simulink model "ssc_airvtol_elec_battery"  (R2026a)
settings: Solver=daessc  StopTime=2000  AbsTol=1e-3  EnableMultiTasking=on
PreLoadFcn:
  | ssc_airvtol_elec_default_params
  | battery_capacity = 180;battery_pdensity = 240;payload_mass_workspace = 80;
PostLoadFcn:
  | warning('off','physmod:common:gl:sli:rtp:InvalidNonValueReference');
  | warning off Simulink:Engine:SortDiscontinuityInAlgLoop
model workspace (MATLAB code in the model file):
  | v0                 = 0; % Initial vehicle speed
  | wheel_radius = 0.15; % Wheel radius
  | k                   = 1e-2; % Motor losses (W/(N*M)^2)
  | t_torque        = 0.02; % Electric motor time constant
  | rpm0             = 2000; % Engine initial speed demand
undefined symbols (not defined in the file): battery_vnom, propeller_num
libraries: fl_lib x49, nesl_utility x13, ee_lib x12, ssc_airvtol_components x11, sdl_lib x8, simulink x6, batteryecm_lib x2, pack_5p48s8p_Thr_library x2, pack_5p48s8p_1g10g1_5g1g5_Thr_library x1, pack_5p48s8p_1g10g1_Iso_library x1, pack_5p48s8p_1g10g1_Thr_library x1, pack_5p48s8p_4g4g4_Iso_library x1
(part 1 of 2)
CloseFcn:
  | try,close(h1_ssc_airvtol_elec),end
  | clear h1_ssc_airvtol_elec
  | try,close(h2_ssc_airvtol_elec),end
  | clear h2_ssc_airvtol_elec
  | try,close(h3_ssc_airvtol_elec),end
  | clear h3_ssc_airvtol_elec
  | try,close(h4_ssc_airvtol_elec),end
  | clear h4_ssc_airvtol_elec
  | try,close(h5_ssc_airvtol_elec),end
  | clear h5_ssc_airvtol_elec
  | try,close(h6_ssc_airvtol_elec),end
  | clear h6_ssc_airvtol_elec
  | try,close(h7_ssc_airvtol_elec),end
  | clear h7_ssc_airvtol_elec
  | try,close(h8_ssc_airvtol_elec),end
  | clear h8_ssc_airvtol_elec
  | try,close(h9_ssc_airvtol_elec),end
  | clear h9_ssc_airvtol_elec
  | try,close(h10_ssc_airvtol_elec),end
  | clear h10_ssc_airvtol_elec
  | 
  | clear simlog_ssc_airvtol_elec
  | clear logsout_ssc_airvtol_elec
Description:
  | Electric Aircraft (VTOL) Battery Design Exploration
  | 
  | Copyright 2022-2026 The MathWorks, Inc.
settings Model: FPTRunName=Active  Creator=MathWorks  LastModifiedBy=smiller
settings DataIOCC: InitialState=xBaseline  SaveOperatingPoint=on  SignalLoggingSaveFormat=ModelDataLogs  SignalLoggingName=logsout_ssc_airvtol_elec
settings DebuggingCC: UnderspecifiedInitializationDetection=Classic  PregeneratedLibrarySubsystemCodeDiagnostic=none
settings HardwareCC: ProdHWDeviceType=32-bit Generic
settings GRTTargetCC: CombineOutputUpdateFcns=off  GRTInterface=on
settings SimscapeCC: SimscapeNormalizeSystem=off  SimscapeNominalValues="[{\"value\":\"1\",\"unit\":\"A\"},{\"value\":\"1\",\"unit\":\"bar\"},{\"value\":\"1\",\"unit\":\"cm^2\"},{\"value\":\"1\",\"unit\":\"cm^3/s\"},{\"value\":\"1\",\"unit\":\"kJ/kg\"},{\"value\":\"1\",\"unit\":\"kW\"},{\"value\":\"1\",\"unit\":\"l\"},{\"value\":\"1\",\"unit\":\"N\"},{\"value\":\"1\",\"unit\":\"N*m\"},{\"value\":\"1\",\"unit\":\"V\"}]"  SimscapeLogSimulationStatistics=on  SimscapeLogName=simlog_ssc_airvtol_elec

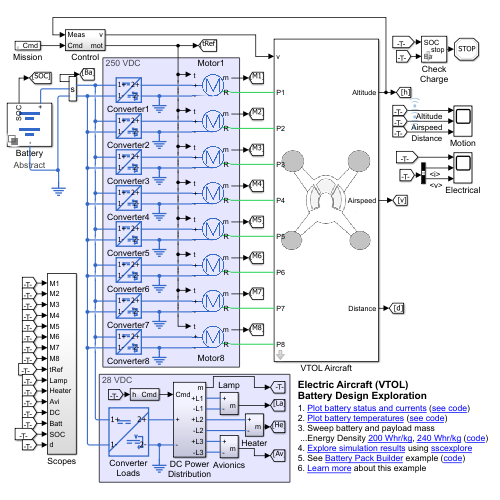
[thumbnail: Simulink's stored preview of the top-level diagram]
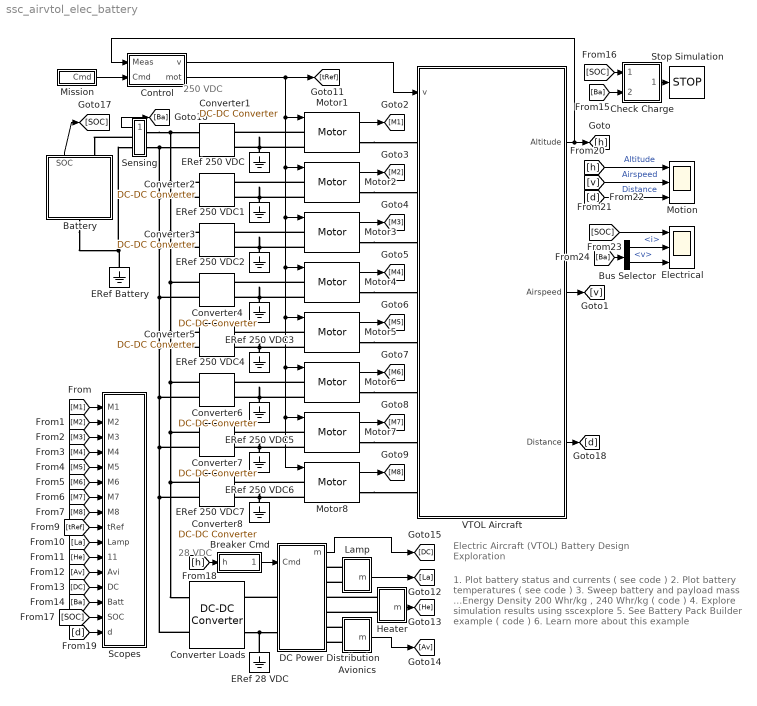
== system ssc_airvtol_elec_battery ==
  note: 250 VDC
  note: 28 VDC
  note: Electric Aircraft (VTOL)
      | Battery Design Exploration
  note: 1. Plot battery status and currents ( see code )
      | 2. Plot battery temperatures ( see code )
      | 3. Sweep battery and payload mass
      | ...Energy Density 200 Whr/kg , 240 Whr/kg ( code )
      | 4. Explore simulation results using sscexplore
      | 5. See Battery Pack Builder example ( code )
      | 6. Learn more about this example
  Avionics : Subsystem
  Battery : Subsystem  Variant=on  VariantControlMode=label  VariantControl=Equal_Iso  LabelModeActiveChoice=Abstract
      settings: AttributesFormatString=%<LabelModeActiveChoice>
  Breaker Cmd : Subsystem
  Bus Selector : BusSelector  OutputSignals=i,v
  Check Charge : Subsystem  mask{q_battery_limit=0.3}
      mask prompts: q_battery_limit "Battery charge lower limit (A*hr)"
  Control : Subsystem
  Converter Loads : ee_lib/Semiconductors & Converters/Converters/DC-DC Converter  Vref_option=ee.enum.converters.voltageref.internal  v_ref=28 V  P_rated=4 kW  droop_enabled=true  droop_param=ee.enum.converters.droop.value  droop=0.01 V/A  droop_percent=2  Vref_droop=10 V  reversible=ee.enum.converters.directionality.unidirectional  G_diode=1e-8 1/Ohm  P_fixed=100 W  losses_option=ee.enum.converters.lossesOption.proportionalToSquaredCurrent  eff_rated=97  tableOption=ee.enum.converters.lossTableOption.current  i_eff_vec=[1, 2, 3, 4] A  v_eff_vec=[15, 30, 45] V  eff_vec=[90, 80, 70, 60]  eff_2D_table=[90, 85, 80; 80, 75, 70; 70, 65, 60; 60, 55, 50]  model_dynamics=ee.enum.converters.dynamics.yes  tau=0.02 s  v_ini=28 V  v1_min=1 V  R1=1000 Ohm  R2=1000 Ohm  T_eff_vec=[280, 300, 320] K  eff_3D_table=repmat([66; 76; 80; 74], 1, 3, 3)  thermal_mass=100 J/K  initial_temperature=298.15 K
  Converter{1..8} (8 alike) : ee_lib/Semiconductors & Converters/Converters/DC-DC Converter  Vref_option=ee.enum.converters.voltageref.internal  v_ref=250 V  P_rated=1200 kW  droop_enabled=true  droop_param=ee.enum.converters.droop.value  droop=0.001 V/A  droop_percent=2  Vref_droop=10 V  reversible=ee.enum.converters.directionality.bidirectional  G_diode=1e-8 1/Ohm  P_fixed=100 W  losses_option=ee.enum.converters.lossesOption.proportionalToSquaredCurrent  eff_rated=97  tableOption=ee.enum.converters.lossTableOption.current  i_eff_vec=[1, 2, 3, 4] A  v_eff_vec=[15, 30, 45] V  eff_vec=[90, 80, 70, 60]  eff_2D_table=[90, 85, 80; 80, 75, 70; 70, 65, 60; 60, 55, 50]  model_dynamics=ee.enum.converters.dynamics.yes  tau=0.02 s  v_ini=250 V  v1_min=1 V  R1=1000 Ohm  R2=1000 Ohm  T_eff_vec=[280, 300, 320] K  eff_3D_table=repmat([66; 76; 80; 74], 1, 3, 3)  thermal_mass=100 J/K  initial_temperature=298.15 K
  DC Power Distribution : Subsystem
  ERef 250 VDC{,1..7} (8 alike) : fl_lib/Electrical/Electrical Elements/Electrical Reference
  ERef 28 VDC : fl_lib/Electrical/Electrical Elements/Electrical Reference
  ERef Battery : fl_lib/Electrical/Electrical Elements/Electrical Reference
  Electrical : Scope  NumInputPorts=3
      settings: Title=Battery SOC  ActiveDisplayYMinimum=0.2125  ActiveDisplayYMaximum=1.0875  DataLoggingVariableName=ScopeData3
  Heater : Subsystem
  Lamp : Subsystem
  Mission : Subsystem  mask(Mission Parameters){t_climb=30, h_cruise=100}
      mask prompts: t_climb "Time to reach cruise height (sec)"; h_cruise "Cruise height (m)"
      mask help: Define mission parameters.
  Motion : Scope  NumInputPorts=3
      settings: ActiveDisplayYMinimum=-12.74881  ActiveDisplayYMaximum=114.73236
  Motor{1..8} (8 alike) : ssc_airvtol_components/Motor  SystemSampleTime=-1  VariantActivationTime=update diagram  EmptyChoice=off  PassThrough=off  PassThroughVariantControl=(default)  EmptyChoiceVariantControl=(default)  AllowFlexibleInterface=on  Latency=0  AutoFrameSizeCalculation=off
  Scopes : Subsystem
  Sensing : Subsystem
      mask Display: disp('s');
  Stop Simulation : Stop
  VTOL Aircraft : Subsystem  mask(VTOL Aircraft){battery_power_density=battery_pdensity, battery_voltage=battery_vnom, battery_capacity=battery_capacity, aircraft_mass=60, inertia_prop=0.09, D_prop=1.5, kt_const=0.15, kp_const=0.13, rho=1.225}
      mask prompts: battery_power_density "Power Density (W*hr/kg)"; battery_voltage "Voltage (V)"; battery_capacity "Capacity (A*hr)"; aircraft_mass "Chassis Mass (without battery) (kg)"; inertia_prop "Inertia (kg*m^2)"; D_prop "Diameter"; kt_const "Thrust coefficient, kT"; kp_const "Power coefficient, kP"; rho "Fluid density"
      mask help: Define parameters for airframe, including values to compute total mass and propeller characteristics.
      mask init:
      | battery_mass = battery_capacity*battery_voltage/battery_power_density;
      mask TypeOptions inertia_prop: Inertia1/inertia | Inertia2/inertia | Inertia3/inertia | Inertia4/inertia | Inertia5/inertia | Inertia6/inertia | Inertia7/inertia | Inertia8/inertia
      mask TypeOptions D_prop: Propeller 1/D | Propeller 2/D | Propeller 3/D | Propeller 4/D | Propeller 5/D | Propeller 6/D | Propeller 7/D | Propeller 8/D
      mask TypeOptions kt_const: Propeller 1/kt_const | Propeller 2/kt_const | Propeller 3/kt_const | Propeller 4/kt_const | Propeller 5/kt_const | Propeller 6/kt_const | Propeller 7/kt_const | Propeller 8/kt_const
      mask TypeOptions kp_const: Propeller 1/kp_const | Propeller 2/kp_const | Propeller 3/kp_const | Propeller 4/kp_const | Propeller 5/kp_const | Propeller 6/kp_const | Propeller 7/kp_const | Propeller 8/kp_const
      mask TypeOptions rho: Propeller 1/rho | Propeller 2/rho | Propeller 3/rho | Propeller 4/rho | Propeller 5/rho | Propeller 6/rho | Propeller 7/rho | Propeller 8/rho
      mask DialogControl Container4 Prompt: Electrical
      mask DialogControl Container5 Prompt: Mechanical
      mask DialogControl cont_prop Prompt: Propeller
      mask Display: image('ssc_airvtol_battery_chassis_IMAGE.png')
  wires:
  VTOL Aircraft/3(Distance) -> [d]
  Breaker Cmd/1(Cmd) -> DC Power Distribution/1(Cmd)
  Check Charge/1(stop) -> Stop Simulation/1
  Battery/1(SOC) -> [SOC]
  VTOL Aircraft/1(Altitude) -> Control/1(Meas), [h]
  Motor1/1 -> [M1]
  Motor2/1 -> [M2]
  Motor3/1 -> [M3]
  Motor4/1 -> [M4]
  Motor5/1 -> [M5]
  Motor6/1 -> [M6]
  Motor7/1 -> [M7]
  Motor8/1 -> [M8]
  Mission/1(Cmd) -> Control/2(Cmd)
  Control/2(mot) -> Motor8/1, Motor7/1, Motor6/1, Motor5/1, Motor4/1, Motor3/1, Motor2/1, Motor1/1, [tRef]
  Control/1(v) -> VTOL Aircraft/1(v)
  [M1] -> Scopes/1(M1)
  [M2] -> Scopes/2(M2)
  [M3] -> Scopes/3(M3)
  [M4] -> Scopes/4(M4)
  [M5] -> Scopes/5(M5)
  [M6] -> Scopes/6(M6)
  [M7] -> Scopes/7(M7)
  [M8] -> Scopes/8(M8)
  [tRef] -> Scopes/9(tRef)
  Lamp/1(m) -> [La]
  [La] -> Scopes/10(Lamp)
  Heater/1(m) -> [He]
  Avionics/1(m) -> [Av]
  [He] -> Scopes/11(Heater)
  [Av] -> Scopes/12(Avi)
  DC Power Distribution/1(m) -> [DC]
  [DC] -> Scopes/13(DC)
  Sensing/1(m) -> [Ba]
  [Ba] -> Scopes/14(Batt)
  [Ba] -> Check Charge/2(Ba)
  [SOC] -> Check Charge/1(SOC)
  [SOC] -> Scopes/15(SOC)
  VTOL Aircraft/2(Airspeed) -> [v]
  [h] -> Breaker Cmd/1(h)
  [h] -> Motion/1  "Altitude"
  [v] -> Motion/2  "Airspeed"
  [d] -> Motion/3  "Distance"
  [SOC] -> Electrical/1
  [Ba] -> Bus Selector/1
  Bus Selector/1 -> Electrical/2  "<i>"
  Bus Selector/2 -> Electrical/3  "<v>"
  [d] -> Scopes/16(d)
  connections:
  Motor1/RConn1 -- VTOL Aircraft/LConn1
  Motor1/LConn1 -- Converter1/RConn1
  DC Power Distribution/LConn1 -- Converter Loads/RConn1
  Heater/LConn1 -- DC Power Distribution/RConn3
  Lamp/LConn2 -- DC Power Distribution/RConn2
  Lamp/LConn1 -- DC Power Distribution/RConn1
  Heater/LConn2 -- DC Power Distribution/RConn4
  Converter Loads/RConn2 -- ERef 28 VDC/LConn1 -- DC Power Distribution/LConn2
  ERef 250 VDC/LConn1 -- Motor1/LConn2 -- Converter1/RConn2
  ERef Battery/LConn1 -- Battery/LConn1 -- Sensing/RConn2
  Avionics/LConn1 -- DC Power Distribution/RConn5
  Avionics/LConn2 -- DC Power Distribution/RConn6
  Sensing/LConn1 -- Converter2/LConn1 -- Converter3/LConn1 -- Converter4/LConn1 -- Converter5/LConn1 -- Converter6/LConn1 -- Converter7/LConn1 -- Converter8/LConn1 -- Converter Loads/LConn1 -- Converter1/LConn1
  Converter Loads/LConn2 -- Sensing/LConn2 -- Converter1/LConn2 -- Converter2/LConn2 -- Converter3/LConn2 -- Converter4/LConn2 -- Converter5/LConn2 -- Converter6/LConn2 -- Converter7/LConn2 -- Converter8/LConn2
  ERef 250 VDC1/LConn1 -- Motor2/LConn2 -- Converter2/RConn2
  Motor2/LConn1 -- Converter2/RConn1
  Motor2/RConn1 -- VTOL Aircraft/LConn2
  ERef 250 VDC2/LConn1 -- Motor3/LConn2 -- Converter3/RConn2
  Motor3/LConn1 -- Converter3/RConn1
  Motor3/RConn1 -- VTOL Aircraft/LConn3
  ERef 250 VDC3/LConn1 -- Motor4/LConn2 -- Converter4/RConn2
  Motor4/LConn1 -- Converter4/RConn1
  Motor4/RConn1 -- VTOL Aircraft/LConn4
  ERef 250 VDC4/LConn1 -- Motor5/LConn2 -- Converter5/RConn2
  Motor5/LConn1 -- Converter5/RConn1
  Motor5/RConn1 -- VTOL Aircraft/LConn5
  ERef 250 VDC5/LConn1 -- Motor6/LConn2 -- Converter6/RConn2
  Motor6/LConn1 -- Converter6/RConn1
  Motor6/RConn1 -- VTOL Aircraft/LConn6
  ERef 250 VDC6/LConn1 -- Motor7/LConn2 -- Converter7/RConn2
  Motor7/LConn1 -- Converter7/RConn1
  Motor7/RConn1 -- VTOL Aircraft/LConn7
  ERef 250 VDC7/LConn1 -- Motor8/LConn2 -- Converter8/RConn2
  Motor8/LConn1 -- Converter8/RConn1
  Motor8/RConn1 -- VTOL Aircraft/LConn8
  Sensing/RConn1 -- Battery/RConn1

== system ssc_airvtol_elec_battery/Avionics ==
  Electrical Power : ssc_airvtol_components/Motor/Electrical Power  SystemSampleTime=-1  VariantActivationTime=update diagram  EmptyChoice=off  PassThrough=off  PassThroughVariantControl=(default)  EmptyChoiceVariantControl=(default)  AllowFlexibleInterface=on  Latency=0  AutoFrameSizeCalculation=off
  Resistor : fl_lib/Electrical/Electrical Elements/Resistor  R=1.5 Ohm  i_specify=off  i_priority=None  i=0 A  i_nominal_specify=off  i_nominal_value=1  i_nominal_unit=A  v_specify=off  v_priority=None  v=0 V  v_nominal_specify=off  v_nominal_value=1  v_nominal_unit=V
  + : PMIOPort  Side=Left
  - : PMIOPort  Port=2  Side=Left
  Out Bus Element : Outport  PortName=m  Element=Pe
  Out Bus Element3 : Outport  PortName=m  Element=i
  wires:
  Electrical Power/2 -> Out Bus Element3/1
  Electrical Power/1 -> Out Bus Element/1
  connections:
  Electrical Power/LConn1 -- +/RConn1
  Resistor/LConn1 -- Electrical Power/RConn1
  Resistor/RConn1 -- Electrical Power/LConn2 -- -/RConn1

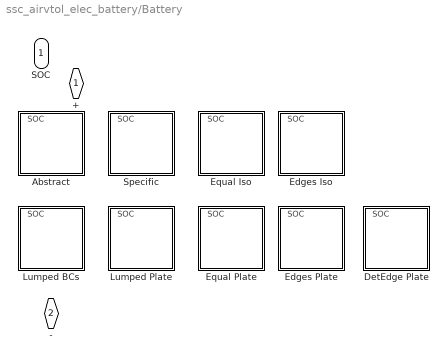
== system ssc_airvtol_elec_battery/Battery ==
  Abstract : Subsystem  VariantControl=Abstract
      mask Display: image('pack_abstract_IMAGE.png');
  DetEdge Plate : Subsystem  VariantControl=DetEdge_Plate
      mask Display: image('pack_5p48s8p_1g10g1_5g1g5_plate_IMAGE.png')
  Edges Iso : Subsystem  VariantControl=Edges_Iso
      mask Display: image('pack_5p48s8p_1g10g1_IMAGE.png')
  Edges Plate : Subsystem  VariantControl=Edges_Plate
      mask Display: image('pack_5p48s8p_1g10g1_plate_IMAGE.png')
  Equal Iso : Subsystem  VariantControl=Equal_Iso
      mask Display: image('pack_5p48s8p_4g4g4_IMAGE.png')
  Equal Plate : Subsystem  VariantControl=Equal_Plate
      mask Display: image('pack_5p48s8p_4g4g4_plate_IMAGE.png')
  Lumped BCs : Subsystem  VariantControl=Lumped_BCs
      mask Display: image('pack_5p48s8p_bcnd_IMAGE.png')
  Lumped Plate : Subsystem  VariantControl=Lumped_Plate
      mask Display: image('pack_5p48s8p_plate_IMAGE.png')
  Specific : Subsystem  VariantControl=Specific
      mask Display: image('pack_specific_IMAGE.png');
  + : PMIOPort  Side=Right
  - : PMIOPort  Port=2  Side=Left
  SOC : Outport

== system ssc_airvtol_elec_battery/Breaker Cmd ==
  h : Inport
  Avionics Breaker : Constant
  Heater Breaker OFF : Constant  Value=0
  Heater Breaker ON : Constant
  Lamp Breaker : Constant
  Mux1 : Mux  Inputs=3
  Switch : Switch  Threshold=50  ZeroCross=off  SaturateOnIntegerOverflow=off  InputSameDT=off
  Cmd : Outport  VectorParamsAs1DForOutWhenUnconnected=off
  wires:
  Mux1/1 -> Cmd/1
  Avionics Breaker/1 -> Mux1/3
  Lamp Breaker/1 -> Mux1/1
  Switch/1 -> Mux1/2
  h/1 -> Switch/2
  Heater Breaker ON/1 -> Switch/1
  Heater Breaker OFF/1 -> Switch/3

== system ssc_airvtol_elec_battery/Check Charge ==
  SOC : Inport
  In Bus Element : Inport  Port=2  PortName=Ba  Element=v
  In Bus Element1 : Inport  Port=2  PortName=Ba  Element=i
  Compare To Constant : simulink/Logic and Bit Operations/Compare To Constant  relop=<=  const=q_battery_limit  OutDataTypeStr=boolean
  Compare To Constant1 : simulink/Logic and Bit Operations/Compare To Constant  relop=<=  const=100  OutDataTypeStr=boolean
  Compare To Constant2 : simulink/Logic and Bit Operations/Compare To Constant  relop=>=  const=1000  OutDataTypeStr=boolean
  OR : Logic  Operator=OR  Inputs=3  IconShape=distinctive  AllPortsSameDT=off  OutDataTypeStr=boolean
  stop : Outport  VectorParamsAs1DForOutWhenUnconnected=off
  wires:
  Compare To Constant/1 -> OR/3
  In Bus Element/1 -> Compare To Constant1/1
  In Bus Element1/1 -> Compare To Constant2/1
  OR/1 -> stop/1
  Compare To Constant2/1 -> OR/2
  Compare To Constant1/1 -> OR/1
  SOC/1 -> Compare To Constant/1

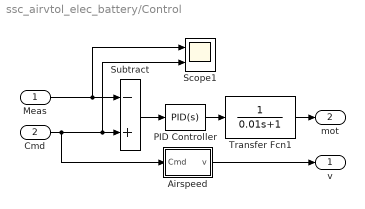
== system ssc_airvtol_elec_battery/Control ==
  Meas : Inport
  Cmd : Inport  Port=2
  Airspeed : Subsystem  mask(Conditions for Cruise){vCruise=28, vzth_Cruise=0.1, zth_Cruise=50}
      mask prompts: vCruise "Cruising speed (m/s)"; vzth_Cruise "Max vertical speed for cruise (m/s)"; zth_Cruise "Min altitude for cruise (m)"
      mask help: Define conditions for cruise speed.
  PID Controller : slpidlib/PID Controller  Controller=PID  Form=Parallel  TimeDomain=Continuous-time  UseExternalTs=off  SampleTime=-1  IntegratorMethod=Forward Euler  FilterMethod=Forward Euler  ControllerParametersSource=internal  P=1*10/2  I=0.08*10  UseKiTs=off  D=0.1*100  UseExternalDerivativeSource=off  N=100/100  UseFilter=on  TunerSelectOption=Transfer Function Based (PID Tuner App)  InitialConditionSource=internal  InitialConditionForIntegrator=0  InitialConditionForFilter=0  DifferentiatorICPrevScaledInput=0  ExternalReset=none  TrackingMode=off  Kt=1  LimitOutput=off  SatLimitsSource=internal  UpperSaturationLimit=inf  LowerSaturationLimit=-inf  LinearizeAsGain=on  AntiWindupMode=none  Kb=1  LimitIntegrator=off  UpperIntegratorSaturationLimit=inf  LowerIntegratorSaturationLimit=-inf  POutMin=[]  POutMax=[]  IOutMin=[]  IOutMax=[]  DOutMin=[]  DOutMax=[]  NOutMin=[]  NOutMax=[]  SumOutMin=[]  SumOutMax=[]  SaturationOutMin=[]  SaturationOutMax=[]  PParamMin=[]  PParamMax=[]  IParamMin=[]  IParamMax=[]  DParamMin=[]  DParamMax=[]  NParamMin=[]  NParamMax=[]  KbParamMin=[]  KbParamMax=[]  KtParamMin=[]  KtParamMax=[]  KbOutMin=[]  KbOutMax=[]  KtOutMin=[]  KtOutMax=[]  IntegratorOutMin=[]  IntegratorOutMax=[]  FilterOutMin=[]  FilterOutMax=[]  SumI1OutMin=[]  SumI1OutMax=[]  SumI2OutMin=[]  SumI2OutMax=[]  SumI3OutMin=[]  SumI3OutMax=[]  SumI4OutMin=[]  SumI4OutMax=[]  SumDOutMin=[]  SumDOutMax=[]  DifferentiatorOutMin=[]  DifferentiatorOutMax=[]  FilterDiffOutCoefMin=[]  FilterDiffOutCoefMax=[]  ReciprocalOutMin=[]  ReciprocalOutMax=[]  SumDenOutMin=[]  SumDenOutMax=[]  SumNumOutMin=[]  SumNumOutMax=[]  DivideOutMin=[]  DivideOutMax=[]  UdiffTsProdOutMin=[]  UdiffTsProdOutMax=[]  NTsProdOutMin=[]  NTsProdOutMax=[]  UintegralTsProdOutMin=[]  UintegralTsProdOutMax=[]  UngainTsProdOutMin=[]  UngainTsProdOutMax=[]  ClampingZeroOutDataTypeStr=Inherit: Inherit via back propagation  ClampingZeroOutMin=[]  ClampingZeroOutMax=[]  FilterDenConstantOutDataTypeStr=Inherit: Inherit via back propagation  FilterDenConstantOutMin=[]  FilterDenConstantOutMax=[]  PCopyOutDataTypeStr=Inherit: Inherit via back propagation  PCopyOutMin=[]  PCopyOutMax=[]  NCopyOutDataTypeStr=Inherit: Inherit via back propagation  NCopyOutMin=[]  NCopyOutMax=[]  IntegratorContinuousStateAttributes=''  IntegratorStateMustResolveToSignalObject=off  IntegratorRTWStateStorageClass=Auto  FilterContinuousStateAttributes=''  FilterStateMustResolveToSignalObject=off  FilterRTWStateStorageClass=Auto  ParallelPVariant=InternalParameters  IdealPVariant=Disabled  IVariant=InternalParameters  DVariant=InternalParameters  IntegratorVariant=Continuous  SatVariant=Disabled  AWVariant=Passthrough  PCopyVariant=Disabled  TRVariant=Disabled  FdbkBlocksVariant=Forward  IdealPFdbkVariant=Disabled  SatFdbkVariant=Disabled  DerivativeFilterVariant=ContFilter  NVariant=InternalParameters  NCopyVariant=Disabled  FilterICVariant=InternalICsFilter  IntegratorICVariant=InternalICs  ExternalResetVariant=Disabled  TRSumVariant=Passthrough  SumFdbkVariant=Disabled  SumVariant=Sum_PID  TsampFilterVariant=InternalTs  TsampNgainVariant=Passthrough  TsampIntegralVariant=Disabled_SignalSpec  ExternalSaturationOutDataTypeStr=Inherit: Same as second input  DerivativeSourceVariant=ErrorSignal  PreIntVariant=InternalPreInt
  Scope1 : Scope  NumInputPorts=2
      settings: ActiveDisplayYMinimum=-1.70644  ActiveDisplayYMaximum=15.34881
  Subtract : Sum  Inputs=-+
  Transfer Fcn1 : TransferFcn  Denominator=[0.01 1]
  v : Outport
  mot : Outport  Port=2
  wires:
  Subtract/1 -> PID Controller/1
  PID Controller/1 -> Transfer Fcn1/1
  Transfer Fcn1/1 -> mot/1
  Cmd/1 -> Airspeed/1(Cmd), Scope1/2, Subtract/2
  Meas/1 -> Scope1/1, Subtract/1
  Airspeed/1(v) -> v/1

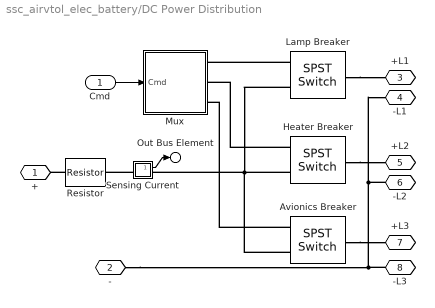
== system ssc_airvtol_elec_battery/DC Power Distribution ==
  Cmd : Inport
  Avionics Breaker : ee_lib/Switches & Breakers/SPST Switch  R_closed=0.001 Ohm  G_open=1e-3 S  Threshold=0.5 V  Width=0 V  model_dynamics=0  t_on=1e-3 s  t_off=1e-3 s  initial_vT=0 V
  Heater Breaker : ee_lib/Switches & Breakers/SPST Switch  R_closed=0.001 Ohm  G_open=1e-3 S  Threshold=0.5 V  Width=0 V  model_dynamics=0  t_on=1e-3 s  t_off=1e-3 s  initial_vT=0 V
  Lamp Breaker : ee_lib/Switches & Breakers/SPST Switch  R_closed=0.001 Ohm  G_open=1e-3 S  Threshold=0.5 V  Width=0 V  model_dynamics=0  t_on=1e-3 s  t_off=1e-3 s  initial_vT=0 V
  Mux : Subsystem
  Resistor : fl_lib/Electrical/Electrical Elements/Resistor  R=0.002 Ohm  i_specify=off  i_priority=None  i=0 A  i_nominal_specify=off  i_nominal_value=1  i_nominal_unit=A  v_specify=off  v_priority=None  v=0 V  v_nominal_specify=off  v_nominal_value=1  v_nominal_unit=V
  Sensing Current : Subsystem
      mask Display: disp('i')
  + : PMIOPort  Side=Left
  - : PMIOPort  Port=2  Side=Left
  +L1 : PMIOPort  Port=3  Side=Right
  -L1 : PMIOPort  Port=4  Side=Right
  +L2 : PMIOPort  Port=5  Side=Right
  -L2 : PMIOPort  Port=6  Side=Right
  +L3 : PMIOPort  Port=7  Side=Right
  -L3 : PMIOPort  Port=8  Side=Right
  Out Bus Element : Outport  PortName=m  Element=i
  wires:
  Cmd/1 -> Mux/1(Cmd)
  Sensing Current/1(i) -> Out Bus Element/1
  connections:
  Heater Breaker/LConn2 -- Lamp Breaker/LConn2 -- Sensing Current/RConn1 -- Avionics Breaker/LConn2
  -/RConn1 -- -L3/RConn1 -- -L2/RConn1 -- -L1/RConn1
  Lamp Breaker/RConn1 -- +L1/RConn1
  Heater Breaker/RConn1 -- +L2/RConn1
  Avionics Breaker/RConn1 -- +L3/RConn1
  Resistor/LConn1 -- +/RConn1
  Lamp Breaker/LConn1 -- Mux/RConn1
  Heater Breaker/LConn1 -- Mux/RConn2
  Avionics Breaker/LConn1 -- Mux/RConn3
  Sensing Current/LConn1 -- Resistor/RConn1

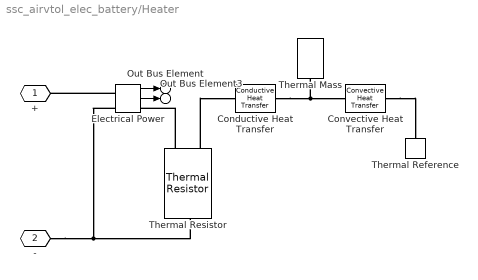
== system ssc_airvtol_elec_battery/Heater ==
  Conductive Heat Transfer : fl_lib/Thermal/Thermal Elements/Conductive Heat Transfer  thermal_type=foundation.enum.ConstantVariableTabulated.Constant  wall_geometry=foundation.enum.ConductionWallGeometry.Planar  area=1e-4 m^2  thickness=0.1 m  d_in=0.05 m  d_out=0.1 m  L=1 m  th_cond_min=10 W/(K*m)  th_cond=401 W/(m*K)  th_cond_TLU=[413, 401, 392, 383, 371, 357, 342] W/(K*m)  temp_TLU=[200, 273, 400, 600, 800, 1000, 1200] K  T_specify=off  T_priority=None  T=0 K  T_nominal_specify=off  T_nominal_value=1  T_nominal_unit=K  Q_specify=off  Q_priority=None  Q=0 J/s  Q_nominal_specify=off  Q_nominal_value=1  Q_nominal_unit=J/s
  Convective Heat Transfer : fl_lib/Thermal/Thermal Elements/Convective Heat Transfer  thermal_type=foundation.enum.constant_variable.constant  area=1e-4 m^2  heat_tr_coeff=20 W/(m^2 * K)  min_heat_tr_coeff=1e-3 W/(K*m^2)  T_specify=off  T_priority=None  T=0 K  T_nominal_specify=off  T_nominal_value=1  T_nominal_unit=K  Q_specify=off  Q_priority=None  Q=0 J/s  Q_nominal_specify=off  Q_nominal_value=1  Q_nominal_unit=J/s
  Electrical Power : ssc_airvtol_components/Motor/Electrical Power  SystemSampleTime=-1  VariantActivationTime=update diagram  EmptyChoice=off  PassThrough=off  PassThroughVariantControl=(default)  EmptyChoiceVariantControl=(default)  AllowFlexibleInterface=on  Latency=0  AutoFrameSizeCalculation=off
  Thermal Mass : fl_lib/Thermal/Thermal Elements/Thermal Mass  mass_type=foundation.enum.constant_variable.constant  mass=1 kg  sp_heat=447 J/kg/K  mass_min=1e-6 kg  num_ports=foundation.enum.numPorts2.one  m_specify=off  m_priority=High  m=1 kg  m_nominal_specify=off  m_nominal_value=1  m_nominal_unit=kg  T_specify=on  T_priority=High  T=300 K  T_nominal_specify=off  T_nominal_value=1  T_nominal_unit=K  Q_specify=off  Q_priority=None  Q=0 J/s  Q_nominal_specify=off  Q_nominal_value=1  Q_nominal_unit=J/s
  Thermal Reference : fl_lib/Thermal/Thermal Elements/Thermal Reference
  Thermal Resistor : fl_lib/Electrical/Electrical Elements/Thermal Resistor  R0=1 Ohm  T0=25 degC  alpha=5e-5 1/K  thermalMassParameterization=foundation.enum.ThermalMassParameterization.TimeConstantAndDissipationFactor  mass=2.6316e-5 kg  cp=380 J/(K*kg)  tc=10 s  K_d=1e-3 W/K  T_specify=on  T_priority=High  T=300 K  T_nominal_specify=off  T_nominal_value=1  T_nominal_unit=K
  + : PMIOPort  Side=Left
  - : PMIOPort  Port=2  Side=Left
  Out Bus Element : Outport  PortName=m  Element=Pe
  Out Bus Element3 : Outport  PortName=m  Element=i
  wires:
  Electrical Power/1 -> Out Bus Element/1
  Electrical Power/2 -> Out Bus Element3/1
  connections:
  Thermal Resistor/LConn2 -- Electrical Power/RConn1
  Conductive Heat Transfer/RConn1 -- Convective Heat Transfer/LConn1 -- Thermal Mass/LConn1
  Thermal Resistor/LConn1 -- Conductive Heat Transfer/LConn1
  Convective Heat Transfer/RConn1 -- Thermal Reference/LConn1
  -/RConn1 -- Electrical Power/LConn2 -- Thermal Resistor/RConn1
  Electrical Power/LConn1 -- +/RConn1

== system ssc_airvtol_elec_battery/Lamp ==
  Electrical Power : ssc_airvtol_components/Motor/Electrical Power  SystemSampleTime=-1  VariantActivationTime=update diagram  EmptyChoice=off  PassThrough=off  PassThroughVariantControl=(default)  EmptyChoiceVariantControl=(default)  AllowFlexibleInterface=on  Latency=0  AutoFrameSizeCalculation=off
  Resistor : fl_lib/Electrical/Electrical Elements/Resistor  R=1 Ohm  i_specify=off  i_priority=High  i=0 A  i_nominal_specify=off  i_nominal_value=1  i_nominal_unit=A  v_specify=off  v_priority=None  v=0 V  v_nominal_specify=off  v_nominal_value=1  v_nominal_unit=V
  + : PMIOPort  Side=Left
  - : PMIOPort  Port=2  Side=Left
  Out Bus Element : Outport  PortName=m  Element=Pe
  Out Bus Element3 : Outport  PortName=m  Element=i
  wires:
  Electrical Power/1 -> Out Bus Element/1
  Electrical Power/2 -> Out Bus Element3/1
  connections:
  -/RConn1 -- Electrical Power/LConn2 -- Resistor/RConn1
  Resistor/LConn1 -- Electrical Power/RConn1
  Electrical Power/LConn1 -- +/RConn1

== system ssc_airvtol_elec_battery/Mission ==
  Height : simulink/Sources/Ramp  slope=h_cruise/t_climb  start=1  InitialOutput=0
  Limits : Saturate  UpperLimit=h_cruise  ZeroCross=off
  Transfer Fcn : TransferFcn  Denominator=[1 1]
  Cmd : Outport
  wires:
  Limits/1 -> Transfer Fcn/1
  Height/1 -> Limits/1
  Transfer Fcn/1 -> Cmd/1

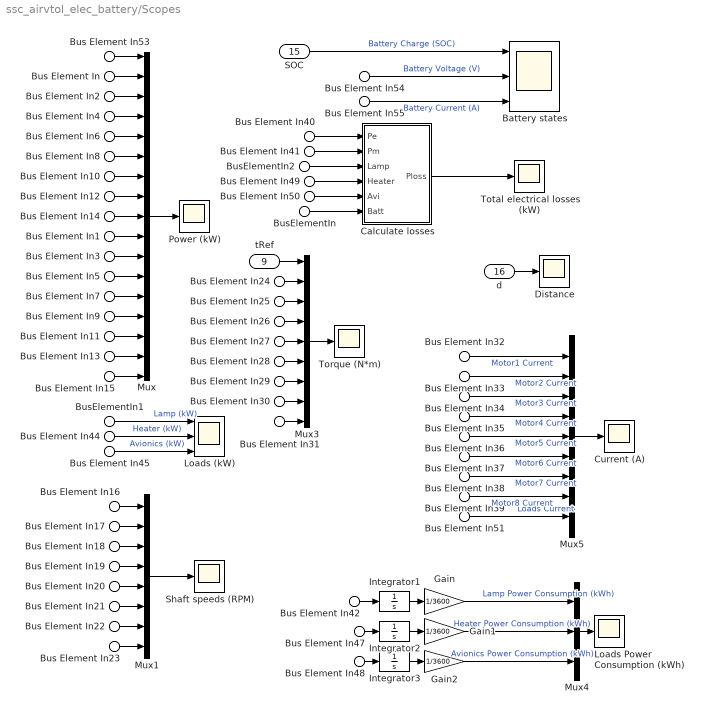
== system ssc_airvtol_elec_battery/Scopes ==
  Bus Element In : Inport  PortName=M1  Element=Pe
  Bus Element In40 : Inport  PortName=M1  Element=Pe
  Bus Element In1 : Inport  PortName=M1  Element=Pm
  Bus Element In41 : Inport  PortName=M1  Element=Pm
  Bus Element In16 : Inport  PortName=M1  Element=w
  Bus Element In24 : Inport  PortName=M1  Element=trq
  Bus Element In32 : Inport  PortName=M1  Element=i
  Bus Element In2 : Inport  Port=2  PortName=M2  Element=Pe
  Bus Element In3 : Inport  Port=2  PortName=M2  Element=Pm
  Bus Element In17 : Inport  Port=2  PortName=M2  Element=w
  Bus Element In25 : Inport  Port=2  PortName=M2  Element=trq
  Bus Element In33 : Inport  Port=2  PortName=M2  Element=i
  Bus Element In4 : Inport  Port=3  PortName=M3  Element=Pe
  Bus Element In5 : Inport  Port=3  PortName=M3  Element=Pm
  Bus Element In18 : Inport  Port=3  PortName=M3  Element=w
  Bus Element In26 : Inport  Port=3  PortName=M3  Element=trq
  Bus Element In34 : Inport  Port=3  PortName=M3  Element=i
  Bus Element In6 : Inport  Port=4  PortName=M4  Element=Pe
  Bus Element In7 : Inport  Port=4  PortName=M4  Element=Pm
  Bus Element In19 : Inport  Port=4  PortName=M4  Element=w
  Bus Element In27 : Inport  Port=4  PortName=M4  Element=trq
  Bus Element In35 : Inport  Port=4  PortName=M4  Element=i
  Bus Element In8 : Inport  Port=5  PortName=M5  Element=Pe
  Bus Element In9 : Inport  Port=5  PortName=M5  Element=Pm
  Bus Element In20 : Inport  Port=5  PortName=M5  Element=w
  Bus Element In28 : Inport  Port=5  PortName=M5  Element=trq
  Bus Element In36 : Inport  Port=5  PortName=M5  Element=i
  Bus Element In10 : Inport  Port=6  PortName=M6  Element=Pe
  Bus Element In11 : Inport  Port=6  PortName=M6  Element=Pm
  Bus Element In21 : Inport  Port=6  PortName=M6  Element=w
  Bus Element In29 : Inport  Port=6  PortName=M6  Element=trq
  Bus Element In37 : Inport  Port=6  PortName=M6  Element=i
  Bus Element In12 : Inport  Port=7  PortName=M7  Element=Pe
  Bus Element In13 : Inport  Port=7  PortName=M7  Element=Pm
  Bus Element In22 : Inport  Port=7  PortName=M7  Element=w
  Bus Element In30 : Inport  Port=7  PortName=M7  Element=trq
  Bus Element In38 : Inport  Port=7  PortName=M7  Element=i
  Bus Element In14 : Inport  Port=8  PortName=M8  Element=Pe
  Bus Element In15 : Inport  Port=8  PortName=M8  Element=Pm
  Bus Element In23 : Inport  Port=8  PortName=M8  Element=w
  Bus Element In31 : Inport  Port=8  PortName=M8  Element=trq
  Bus Element In39 : Inport  Port=8  PortName=M8  Element=i
  tRef : Inport  Port=9
  BusElementIn1 : Inport  Port=10  PortName=Lamp  Element=Pe
  BusElementIn2 : Inport  Port=10  PortName=Lamp  Element=Pe
  Bus Element In{42,44,47,49} (4 alike) : Inport  Port=11  PortName=Heater  Element=Pe
  Bus Element In45 : Inport  Port=12  PortName=Avi  Element=Pe
  Bus Element In48 : Inport  Port=12  PortName=Avi  Element=Pe
  Bus Element In50 : Inport  Port=12  PortName=Avi  Element=Pe
  Bus Element In51 : Inport  Port=13  PortName=DC  Element=i
  BusElementIn : Inport  Port=14  PortName=Batt
  Bus Element In53 : Inport  Port=14  PortName=Batt  Element=Pe
  Bus Element In54 : Inport  Port=14  PortName=Batt  Element=v
  Bus Element In55 : Inport  Port=14  PortName=Batt  Element=i
  SOC : Inport  Port=15
  d : Inport  Port=16
  Battery states : Scope  NumInputPorts=3
      settings: ActiveDisplayYMinimum=0.99644  ActiveDisplayYMaximum=1.0004  DataLoggingVariableName=PureElecBatteryScopeData
  Calculate losses : Subsystem
  Current (A) : Scope
      settings: TimeSpan=20  ActiveDisplayYMinimum=-9.11054  ActiveDisplayYMaximum=81.99488  DataLoggingMaxPoints=50000  DataLoggingVariableName=PureElecCurrentData
  Distance : Scope
      settings: ActiveDisplayYMinimum=-2.90819  ActiveDisplayYMaximum=26.17372  DataLoggingVariableName=Distance  DataLoggingSaveFormat=Array
  Gain : Gain  Gain=1/3600
  Gain1 : Gain  Gain=1/3600
  Gain2 : Gain  Gain=1/3600
  Integrator1 : Integrator
  Integrator2 : Integrator
  Integrator3 : Integrator
  Loads (kW) : Scope  NumInputPorts=3
      settings: ActiveDisplayYMinimum=-0.09715  ActiveDisplayYMaximum=0.8744  DataLoggingMaxPoints=50000
  Loads Power Consumption (kWh) : Scope
      settings: TimeSpan=20  ActiveDisplayYMinimum=-0.00246  ActiveDisplayYMaximum=0.00227  DataLoggingMaxPoints=50000  DataLoggingVariableName=PureElecLoadPowerConsumptionData
  Mux : Mux  Inputs=17
  Mux1 : Mux  Inputs=8
  Mux3 : Mux  Inputs=9
  Mux4 : Mux  Inputs=3
  Mux5 : Mux  Inputs=9
  Power (kW) : Scope
      settings: TimeSpan=20  ActiveDisplayYMinimum=-14.18196  ActiveDisplayYMaximum=127.63764  DataLoggingMaxPoints=50000  DataLoggingVariableName=ScopeData8
  Shaft speeds (RPM) : Scope
      settings: ActiveDisplayYMinimum=-168.98555  ActiveDisplayYMaximum=1520.86993  DataLoggingMaxPoints=50000
  Torque (N*m) : Scope
      settings: TimeSpan=2000  ActiveDisplayYMinimum=-8.29359  ActiveDisplayYMaximum=74.62136  DataLoggingMaxPoints=50000
  Total electrical losses (kW) : Scope
      settings: TimeSpan=20  ActiveDisplayYMinimum=-1.88992  ActiveDisplayYMaximum=29.92464  DataLoggingVariableName=ScopeData3
  wires:
  SOC/1 -> Battery states/1  "Battery Charge (SOC)"
  Calculate losses/1(Ploss) -> Total electrical losses (kW)/1
  Mux1/1 -> Shaft speeds (RPM)/1
  Mux/1 -> Power (kW)/1
  Mux3/1 -> Torque (N*m)/1
  tRef/1 -> Mux3/1
  Bus Element In24/1 -> Mux3/2
  Bus Element In54/1 -> Battery states/2  "Battery Voltage (V)"
  Bus Element In55/1 -> Battery states/3  "Battery Current (A)"
  Bus Element In45/1 -> Loads (kW)/3  "Avionics (kW)"
  Bus Element In44/1 -> Loads (kW)/2  "Heater (kW)"
  Mux4/1 -> Loads Power Consumption (kWh)/1
  Bus Element In47/1 -> Integrator2/1
  Bus Element In48/1 -> Integrator3/1
  Integrator1/1 -> Gain/1
  Gain/1 -> Mux4/1  "Lamp Power Consumption (kWh)"
  Integrator2/1 -> Gain1/1
  Gain1/1 -> Mux4/2  "Heater Power Consumption (kWh)"
  Integrator3/1 -> Gain2/1
  Gain2/1 -> Mux4/3  "Avionics Power Consumption (kWh)"
  Bus Element In32/1 -> Mux5/1  "Motor1 Current"
  Bus Element In51/1 -> Mux5/9  "Loads Current"
  Mux5/1 -> Current (A)/1
  Bus Element In33/1 -> Mux5/2  "Motor2 Current"
  Bus Element In34/1 -> Mux5/3  "Motor3 Current"
  Bus Element In35/1 -> Mux5/4  "Motor4 Current"
  Bus Element In36/1 -> Mux5/5  "Motor5 Current"
  Bus Element In37/1 -> Mux5/6  "Motor6 Current"
  Bus Element In38/1 -> Mux5/7  "Motor7 Current"
  Bus Element In39/1 -> Mux5/8  "Motor8 Current"
  Bus Element In53/1 -> Mux/1
  Bus Element In/1 -> Mux/2
  Bus Element In2/1 -> Mux/3
  Bus Element In4/1 -> Mux/4
  Bus Element In6/1 -> Mux/5
  Bus Element In8/1 -> Mux/6
  Bus Element In10/1 -> Mux/7
  Bus Element In12/1 -> Mux/8
  Bus Element In14/1 -> Mux/9
  Bus Element In1/1 -> Mux/10
  Bus Element In3/1 -> Mux/11
  Bus Element In5/1 -> Mux/12
  Bus Element In7/1 -> Mux/13
  Bus Element In9/1 -> Mux/14
  Bus Element In11/1 -> Mux/15
  Bus Element In13/1 -> Mux/16
  Bus Element In15/1 -> Mux/17
  Bus Element In16/1 -> Mux1/1
  Bus Element In17/1 -> Mux1/2
  Bus Element In18/1 -> Mux1/3
  Bus Element In19/1 -> Mux1/4
  Bus Element In20/1 -> Mux1/5
  Bus Element In21/1 -> Mux1/6
  Bus Element In22/1 -> Mux1/7
  Bus Element In23/1 -> Mux1/8
  Bus Element In25/1 -> Mux3/3
  Bus Element In26/1 -> Mux3/4
  Bus Element In27/1 -> Mux3/5
  Bus Element In28/1 -> Mux3/6
  Bus Element In29/1 -> Mux3/7
  Bus Element In30/1 -> Mux3/8
  Bus Element In31/1 -> Mux3/9
  Bus Element In40/1 -> Calculate losses/1(Pe)
  Bus Element In41/1 -> Calculate losses/2(Pm)
  Bus Element In49/1 -> Calculate losses/4(Heater)
  Bus Element In50/1 -> Calculate losses/5(Avi)
  BusElementIn/1 -> Calculate losses/6(Batt)
  BusElementIn1/1 -> Loads (kW)/1  "Lamp (kW)"
  BusElementIn2/1 -> Calculate losses/3(Lamp)
  Bus Element In42/1 -> Integrator1/1
  d/1 -> Distance/1

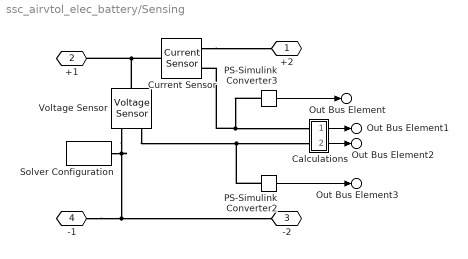
== system ssc_airvtol_elec_battery/Sensing ==
  Calculations : Subsystem
  Current Sensor : fl_lib/Electrical/Electrical Sensors/Current Sensor
  PS-Simulink Converter2 : nesl_utility/PS-Simulink Converter  PhysicalDomain=network_engine_domain  SubClassName=ps_output  LeftPortType=input  RightPortType=output  PseudoPeriodic=off  Frequencies=[]  VectorFormat=1-D array  Unit=V  AffineConversion=off
  PS-Simulink Converter3 : nesl_utility/PS-Simulink Converter  PhysicalDomain=network_engine_domain  SubClassName=ps_output  LeftPortType=input  RightPortType=output  PseudoPeriodic=off  Frequencies=[]  VectorFormat=1-D array  Unit=A  AffineConversion=off
  Solver Configuration : nesl_utility/Solver Configuration  PhysicalDomain=network_engine_domain  SubClassName=solver  LeftPortType=input  RightPortType=generic  Tones=[]  Harmonics=[]  SimulateNoise=off  Profile=off  UseLocalSampling=off  EnableSwitchedLinearOptims=on  FrequencyDomain=off  UseCCode=off  RelTol=0.001  AbsTol=1e-06  MinStep=1e-09  ToWorkspace=off  RevertToSquareIcSolve=off  NumHomotopyIterations=100  PhasorMode=off  PhasorModeNumHarmonics=1  ConsistencySolver=NEWTON_FTOL  CanonicalOrdering=UNORDERED  OptimizeIntermediates=UNOPTIMIZED  IndexReductionMethod=None  DoDC=off  ResidualTolerance=1e-9  ConsistencyTolSource=GLOBAL  ConsistencyAbsTol=0.001  ConsistencyRelTol=0.001  ConsistencyTolFactor=0.001  UseLocalSolver=off  LocalSolverChoice=NE_BACKWARD_EULER_ADVANCER  ResolveIndetEquations=on  FunctionEvalNumThread=1  LocalSolverSampleTime=0.01  DoFixedCost=off  MaxNonlinIter=3  MaxModeIter=2  ComputeImpulses=off  ImpulseIterations=2  LinearAlgebra=Sparse  LinearAlgebraNumThread=0  EquationFormulation=NE_TIME_EF  DelaysMemoryBudget=1024  AutomaticFiltering=on  FilteringTimeConstant=0.001  PartitionStorageMethod=AS_NEEDED  PartitionMemoryBudget=1024  PartitionMethod=FAST  MultibodyUseLocalSolver=off  MultibodyLocalSolverChoice=ODE1  MultibodyLocalSolverSampleTime=0.001
  Voltage Sensor : fl_lib/Electrical/Electrical Sensors/Voltage Sensor
  +2 : PMIOPort  Side=Left
  +1 : PMIOPort  Port=2  Side=Right
  -2 : PMIOPort  Port=3  Side=Left
  -1 : PMIOPort  Port=4  Side=Right
  Out Bus Element : Outport  PortName=m  Element=i
  Out Bus Element1 : Outport  PortName=m  Element=Pe
  Out Bus Element2 : Outport  PortName=m  Element=Po
  Out Bus Element3 : Outport  PortName=m  Element=v
  wires:
  PS-Simulink Converter2/1 -> Out Bus Element3/1
  PS-Simulink Converter3/1 -> Out Bus Element/1
  Calculations/1(Pe) -> Out Bus Element1/1
  Calculations/2(Po) -> Out Bus Element2/1
  connections:
  Current Sensor/RConn2 -- +2/RConn1
  PS-Simulink Converter3/LConn1 -- Calculations/LConn1 -- Current Sensor/RConn1
  Voltage Sensor/RConn1 -- PS-Simulink Converter2/LConn1 -- Calculations/LConn2
  Current Sensor/LConn1 -- +1/RConn1 -- Voltage Sensor/LConn1
  Voltage Sensor/RConn2 -- Solver Configuration/RConn1 -- -1/RConn1 -- -2/RConn1

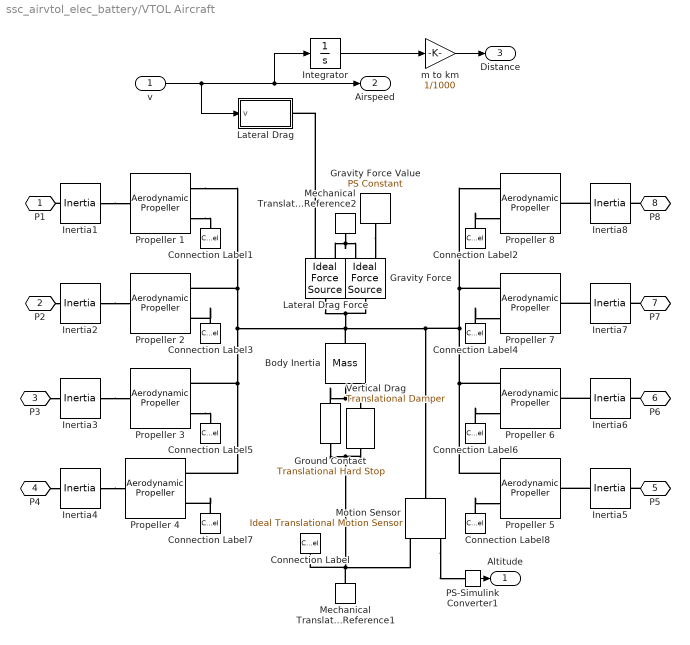
== system ssc_airvtol_elec_battery/VTOL Aircraft ==
  v : Inport
  Body Inertia : fl_lib/Mechanical/Translational Elements/Mass  mass=payload_mass_workspace+battery_mass+aircraft_mass kg  num_ports=foundation.enum.numPorts2.two  v_specify=off  v_priority=High  v=0 m/s  v_nominal_specify=off  v_nominal_value=1  v_nominal_unit=m/s  f_specify=off  f_priority=None  f=0 N  f_nominal_specify=off  f_nominal_value=1  f_nominal_unit=N
  Connection Label{,1..8} (9 alike) : ConnectionLabel  Label=TRef
  Gravity Force : fl_lib/Mechanical/Mechanical Sources/Ideal Force Source
  Gravity Force Value : fl_lib/Physical Signals/Sources/PS Constant  constant=-(payload_mass_workspace+battery_mass+aircraft_mass)*9.81 N
  Ground Contact : fl_lib/Mechanical/Translational Elements/Translational Hard Stop  upper_bnd=1000 m  lower_bnd=0 m  model=simscape.enum.hardstop.fullundamped  stiff_up=1e6 N/m  stiff_low=1e6*8 N/m  D_up=150 N*s/m  D_low=150*8 N*s/m  transition=0.1 mm  coeff_rest=0.7  v_tol=0.001 m/s  f_tol=0.001 N  v_specify=off  v_priority=None  v=0 m/s  v_nominal_specify=off  v_nominal_value=1  v_nominal_unit=m/s  f_specify=off  f_priority=None  f=0 N  f_nominal_specify=off  f_nominal_value=1  f_nominal_unit=N  x_specify=off  x_priority=High  x=0 m  x_nominal_specify=off  x_nominal_value=1  x_nominal_unit=m  M_specify=off  M_priority=None  M=0
  Inertia{1..8} (8 alike) : fl_lib/Mechanical/Rotational Elements/Inertia  inertia=inertia_prop kg*m^2  num_ports=foundation.enum.numPorts2.two  w_specify=off  w_priority=High  w=0 rpm  w_nominal_specify=off  w_nominal_value=1  w_nominal_unit=rad/s  t_specify=off  t_priority=None  t=0 N*m  t_nominal_specify=off  t_nominal_value=1  t_nominal_unit=N*m
  Integrator : Integrator
  Lateral Drag Force : fl_lib/Mechanical/Mechanical Sources/Ideal Force Source
  Lateral Drag : Subsystem
  Mechanical Translational Reference1 : fl_lib/Mechanical/Translational Elements/Mechanical Translational Reference
  Mechanical Translational Reference2 : fl_lib/Mechanical/Translational Elements/Mechanical Translational Reference
  Motion Sensor : fl_lib/Mechanical/Mechanical Sensors/Ideal Translational Motion Sensor  reference=foundation.enum.MeasurementReference.difference  acceleration_port=false  velocity_port=true  position_port=true  offset=0 m
  PS-Simulink Converter1 : nesl_utility/PS-Simulink Converter  PhysicalDomain=network_engine_domain  SubClassName=ps_output  LeftPortType=input  RightPortType=output  PseudoPeriodic=off  Frequencies=[]  VectorFormat=inherit  Unit=inherit  AffineConversion=off
  Propeller {1..8} (8 alike) : sdl_lib/Engines & Motors/Aerodynamic Propeller  parameterization=sdl.enum.PropellerParameterization.Constant  enable_collective_pitch_control=false  enable_transverse_flow=false  direction=sdl.enum.PropellerDirection.Positive  root_pitch=0 deg  D=D_prop m  kt_const=kt_const  kp_const=kp_const  kt_poly_fixed=[.002, .0006, -.0509, .0617]  kp_poly_fixed=[-.0752, .0577, -.0622, .16]  pitch_angle_TLU=[-15, 15, 25, 35, 45] deg  kt_poly_TLU=[.0002, -.00041, -.036, .03; .00026, -.00056, -.048, .04; .002, .00063, -.051, .062; .0014, -.0016, -.048, .087; .00087, -.0036, -.041, .12]  kp_poly_TLU=[-.1, .031, .0055, .088; -.081, -.025, .0044, .07; -.075, .058, -.062, .16; -.052, .065, -.08, .3; -.031, .057, -.069, .4]  J_TLU=[.01, .3, .625, 1.55, 2, 2.6]  kt_TLU_1D=[.0614, .0473, .0318, -.0127, -.0343, -.063]  kp_TLU_1D=[.1496, .1314, .116, -.0521, -.1503, -.2813]  kt_TLU_2D=[.00019, .013, .0048, -.017, -.03, -.045; .00039, .025, .0096, -.037, -.06, -.09; .00061, .047, .032, -.013, -.034, -.063; .00086, .072, .057, .014, -.0076, -.036; .12, .104, .09, .049, .029, .0019]  kp_TLU_2D=[.029, .029, .016, .06, .009, -.16; .059, .054, .031, -.12, -.19, -.29; .15, .13, .12, -.052, -.15, -.28; .26, .24, .22, .097, -.04, -.25; .39, .39, .38, .32, .24, .062]  beta_TLU=linspace(0, 360, 10) deg  Ct_TLU_1D=0.035 * sind(linspace(0, 360, 10) - 200)  Cq_TLU_1D=0.010 * sind(linspace(0, 360, 10) - 200)  Ct_TLU_2D=[0.01 * sind(linspace(0, 360, 10) - 200); 0.020 * sind(linspace(0, 360, 10) - 200); 0.035 * sind(linspace(0, 360, 10) - 200); 0.04 * sind(linspace(0, 360, 10) - 200); 0.06 * sind(linspace(0, 360, 10) - 200)]  Cq_TLU_2D=[0.0005 * sind(linspace(0, 360, 10) - 200); 0.0015 * sind(linspace(0, 360, 10) - 200); 0.0025 * sind(linspace(0, 360, 10) - 200); 0.0035 * sind(linspace(0, 360, 10) - 200); 0.0045 * sind(linspace(0, 360, 10) - 200)]  n_blades=2  radial_TLU=[.1, .12, .2, .4, .6, .8, 1]  twist_TLU=[30, 35, 50, 30, 20, 15, 10] deg  chord_TLU=[.0676, .0666, .0824, .1025, .0885, .0598, .0133]  alpha_TLU=-180 : 10 : 180 deg  Cl_TLU=[.1326, .1326, .1274, .1274, .1274, .1274, .1274; .3626, .3626, .5002, .5002, .5002, .5002, .5002; .5528, .5528, .8007, .8007, .8007, .8007, .8007; .7256, .7256, 1.0125, 1.0125, 1.0125, 1.0125, 1.0125; .8016, .8016, 1.1556, 1.1556, 1.1556, 1.1556, 1.1556; .7873, .7873, 1.1604, 1.1604, 1.1604, 1.1604, 1.1604; .7031, .7031, 1.0493, 1.0493, 1.0493, 1.0493, 1.0493; .5423, .5423, .7973, .7973, .7973, .7973, .7973; .3537, .3537, .4332, .4332, .4332, .4332, .4332; .1155, .1155, -.0376, -.0376, -.0376, -.0376, -.0376; -.1045, -.1045, -.4096, -.4096, -.4096, -.4096, -.4096; -.2999, -.2999, -.672, -.672, -.672, -.672, -.672; -.4401, -.4401, -.9343, -.9343, -.9343, -.9343, -.9343; -.5186, -.5186, -1.0477, -1.0477, -1.0477, -1.0477, -1.0477; -.5303, -.5303, -1.0387, -1.0387, -1.0387, -1.0387, -1.0387; -.5073, -.5073, -.9565, -.9565, -.9565, -.9565, -.9565; -.442, -.442, -.7713, -.7713, -.7713, -.7713, -.7713; -.2658, -.2658, -.4832, -.4832, -.4832, -.4832, -.4832; .4109, .4109, .3629, .3629, .3629, .3629, .3629; 1.1635, 1.1635, 1.3779, 1.3779, 1.3779, 1.3779, 1.3779; 1.2412, 1.2412, 1.4033, 1.4033, 1.4033, 1.4033, 1.4033; .7434, .7434, 1.3453, 1.3453, 1.3453, 1.3453, 1.3453; .7908, .7908, 1.2862, 1.2862, 1.2862, 1.2862, 1.2862; .7525, .7525, 1.1562, 1.1562, 1.1562, 1.1562, 1.1562; .6722, .6722, .9487, .9487, .9487, .9487, .9487; .5324, .5324, .7047, .7047, .7047, .7047, .7047; .3365, .3365, .382, .382, .382, .382, .382; .0529, .0529, -.0229, -.0229, -.0229, -.0229, -.0229; -.2728, -.2728, -.316, -.316, -.316, -.316, -.316; -.4135, -.4135, -.6195, -.6195, -.6195, -.6195, -.6195; -.5087, -.5087, -.7847, -.7847, -.7847, -.7847, -.7847; -.5342, -.5342, -.8419, -.8419, -.8419, -.8419, -.8419; -.5166, -.5166, -.7658, -.7658, -.7658, -.7658, -.7658; -.4321, -.4321, -.5707, -.5707, -.5707, -.5707, -.5707; -.2864, -.2864, -.3098, -.3098, -.3098, -.3098, -.3098; -.1073, -.1073, -.0893, -.0893, -.0893, -.0893, -.0893; .1326, .1326, .1274, .1274, .1274, .1274, .1274]  Cd_TLU=[.0055, .0055, .3904, .3904, .3904, .3904, .3904; .0774, .0774, .449, .449, .449, .449, .449; .2412, .2412, .5915, .5915, .5915, .5915, .5915; .4342, .4342, .8307, .8307, .8307, .8307, .8307; .679, .679, 1.0909, 1.0909, 1.0909, 1.0909, 1.0909; .9003, .9003, 1.3868, 1.3868, 1.3868, 1.3868, 1.3868; 1.0825, 1.0825, 1.6565, 1.6565, 1.6565, 1.6565, 1.6565; 1.2281, 1.2281, 1.875, 1.875, 1.875, 1.875, 1.875; 1.3205, 1.3205, 2.017, 2.017, 2.017, 2.017, 2.017; 1.3234, 1.3234, 2.0407, 2.0407, 2.0407, 2.0407, 2.0407; 1.2391, 1.2391, 1.9513, 1.9513, 1.9513, 1.9513, 1.9513; 1.0963, 1.0963, 1.7643, 1.7643, 1.7643, 1.7643, 1.7643; .8978, .8978, 1.5048, 1.5048, 1.5048, 1.5048, 1.5048; .6525, .6525, 1.2281, 1.2281, 1.2281, 1.2281, 1.2281; .4203, .4203, .838, .838, .838, .838, .838; .2428, .2428, .5434, .5434, .5434, .5434, .5434; .0951, .0951, .2517, .2517, .2517, .2517, .2517; .0292, .0292, .0698, .0698, .0698, .0698, .0698; .0148, .0148, .0267, .0267, .0267, .0267, .0267; .0808, .0808, .0509, .0509, .0509, .0509, .0509; .2429, .2429, .1561, .1561, .1561, .1561, .1561; .5019, .5019, .3927, .3927, .3927, .3927, .3927; .7217, .7217, .7438, .7438, .7438, .7438, .7438; .9336, .9336, 1.1277, 1.1277, 1.1277, 1.1277, 1.1277; 1.0984, 1.0984, 1.4838, 1.4838, 1.4838, 1.4838, 1.4838; 1.2274, 1.2274, 1.7877, 1.7877, 1.7877, 1.7877, 1.7877; 1.3016, 1.3016, 1.9779, 1.9779, 1.9779, 1.9779, 1.9779; 1.3305, 1.3305, 2.0516, 2.0516, 2.0516, 2.0516, 2.0516; 1.2889, 1.2889, 1.9974, 1.9974, 1.9974, 1.9974, 1.9974; 1.1677, 1.1677, 1.8463, 1.8463, 1.8463, 1.8463, 1.8463; 1.0076, 1.0076, 1.5699, 1.5699, 1.5699, 1.5699, 1.5699; .8068, .8068, 1.2596, 1.2596, 1.2596, 1.2596, 1.2596; .5688, .5688, .9493, .9493, .9493, .9493, .9493; .3604, .3604, .6154, .6154, .6154, .6154, .6154; .1802, .1802, .5015, .5015, .5015, .5015, .5015; .0699, .0699, .4265, .4265, .4265, .4265, .4265; .0055, .0055, .3904, .3904, .3904, .3904, .3904]  interp_method=simscape.enum.interpolation.linear  extrap_method=simscape.enum.extrapolation.linear  n_blade_discretization=20  n_azimuthal_discretization=10  density_spec=foundation.enum.constant_variable.constant  rho=rho kg/m^3  rotational_ports=sdl.enum.ConnectionType.Conserving  translational_ports=sdl.enum.ConnectionType.Conserving  model_inertia=false  propeller_inertia=1 kg*m^2  propeller_mass=10 kg  efficiency_sensor=false  n_thr=0.001 Hz  k_thr=0.001  P_thr=0.01 W  operation_check=simscape.enum.assert.action.warn  expose_port_C=0  w_specify=off  w_priority=None  w=0 rad/s  w_nominal_specify=off  w_nominal_value=1  w_nominal_unit=rad/s  Q_specify=off  Q_priority=None  Q=0 N*m  Q_nominal_specify=off  Q_nominal_value=1  Q_nominal_unit=N*m  v_specify=off  v_priority=None  v=0 m/s  v_nominal_specify=off  v_nominal_value=1  v_nominal_unit=m/s  thrust_specify=off  thrust_priority=None  thrust=0 N  thrust_nominal_specify=off  thrust_nominal_value=1  thrust_nominal_unit=N
  Vertical Drag : fl_lib/Mechanical/Translational Elements/Translational Damper  D=10*8 N*s/m  v_specify=off  v_priority=None  v=0 m/s  v_nominal_specify=off  v_nominal_value=1  v_nominal_unit=m/s  f_specify=off  f_priority=None  f=0 N  f_nominal_specify=off  f_nominal_value=1  f_nominal_unit=N
  m to km : Gain  Gain=1/1000
  P1 : PMIOPort  Side=Left
  P2 : PMIOPort  Port=2  Side=Left
  P3 : PMIOPort  Port=3  Side=Left
  P4 : PMIOPort  Port=4  Side=Left
  P5 : PMIOPort  Port=5  Side=Left
  P6 : PMIOPort  Port=6  Side=Left
  P7 : PMIOPort  Port=7  Side=Left
  P8 : PMIOPort  Port=8  Side=Left
  Altitude : Outport
  Airspeed : Outport  Port=2
  Distance : Outport  Port=3
  wires:
  PS-Simulink Converter1/1 -> Altitude/1
  m to km/1 -> Distance/1
  v/1 -> Lateral Drag/1(v), Airspeed/1, Integrator/1
  Integrator/1 -> m to km/1
  connections:
  Inertia1/LConn1 -- Propeller 1/LConn1
  Inertia1/RConn1 -- P1/RConn1
  Inertia2/LConn1 -- Propeller 2/LConn1
  Inertia3/LConn1 -- Propeller 3/LConn1
  Inertia4/LConn1 -- Propeller 4/LConn1
  Inertia5/LConn1 -- Propeller 5/LConn1
  Inertia6/LConn1 -- Propeller 6/LConn1
  Inertia7/LConn1 -- Propeller 7/LConn1
  Inertia8/LConn1 -- Propeller 8/LConn1
  Body Inertia/LConn1 -- Vertical Drag/LConn1 -- Ground Contact/LConn1
  Gravity Force Value/RConn1 -- Gravity Force/RConn1
  Motion Sensor/RConn3 -- PS-Simulink Converter1/LConn1
  P2/RConn1 -- Inertia2/RConn1
  P3/RConn1 -- Inertia3/RConn1
  P4/RConn1 -- Inertia4/RConn1
  P8/RConn1 -- Inertia8/RConn1
  P7/RConn1 -- Inertia7/RConn1
  P6/RConn1 -- Inertia6/RConn1
  P5/RConn1 -- Inertia5/RConn1
  Propeller 1/RConn1 -- Propeller 2/RConn1 -- Propeller 3/RConn1 -- Propeller 4/RConn1 -- Lateral Drag Force/LConn1 -- Gravity Force/LConn1 -- Propeller 5/RConn1 -- Propeller 6/RConn1 -- Propeller 8/RConn1 -- Propeller 7/RConn1 -- Motion Sensor/LConn1 -- Body Inertia/RConn1
  Mechanical Translational Reference2/LConn1 -- Lateral Drag Force/RConn2 -- Gravity Force/RConn2
  Vertical Drag/RConn1 -- Ground Contact/RConn1 -- Mechanical Translational Reference1/LConn1 -- Connection Label/LConn1 -- Motion Sensor/RConn1
  Propeller 1/RConn2 -- Connection Label1/LConn1
  Connection Label2/LConn1 -- Propeller 8/RConn2
  Connection Label4/LConn1 -- Propeller 7/RConn2
  Connection Label3/LConn1 -- Propeller 2/RConn2
  Propeller 3/RConn2 -- Connection Label5/LConn1
  Connection Label6/LConn1 -- Propeller 6/RConn2
  Connection Label7/LConn1 -- Propeller 4/RConn2
  Connection Label8/LConn1 -- Propeller 5/RConn2
  Lateral Drag Force/RConn1 -- Lateral Drag/RConn1
